simulink model "Enceinte_climatique_sans_correcteur"  (R2025b)
settings: Solver=VariableStepAuto  StartTime=0.0  StopTime=6  RelTol=1e-3
settings Model: Creator=boiteth  LastModifiedBy=rofte

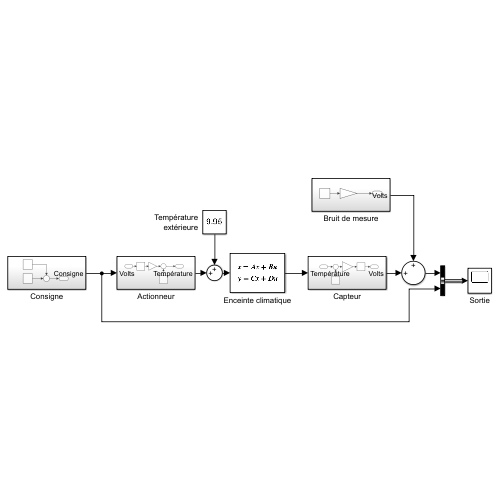
[thumbnail: Simulink's stored preview of the top-level diagram]
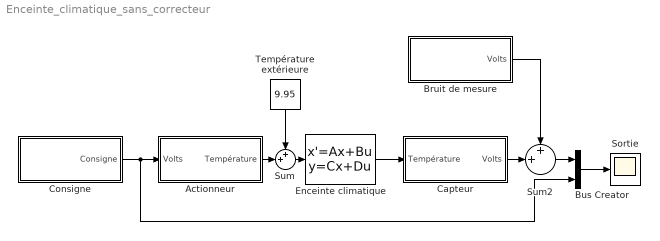
== system Enceinte_climatique_sans_correcteur ==
  Actionneur : Subsystem
  Bruit de mesure : Subsystem
  Bus Creator : BusCreator  Inputs=2
  Capteur : Subsystem
  Consigne : Subsystem
  Enceinte climatique : StateSpace  A=-2  B=2  D=0  InitialCondition=9.95
  Sortie : Scope
      settings: ActiveDisplayYMinimum=-1.1878376392458172  ActiveDisplayYMaximum=6.29146135794454
  Sum : Sum  Inputs=++|
  Sum2 : Sum  Inputs=++|
  Température extérieure : Constant  Value=9.95
  wires:
  Bus Creator/1 -> Sortie/1
  Consigne/1(Consigne) -> Actionneur/1(Volts), Bus Creator/2
  Enceinte climatique/1 -> Capteur/1(Température)
  Actionneur/1(Température) -> Sum/2
  Sum/1 -> Enceinte climatique/1
  Température extérieure/1 -> Sum/1
  Bruit de mesure/1(Volts) -> Sum2/1
  Capteur/1(Volts) -> Sum2/2
  Sum2/1 -> Bus Creator/1

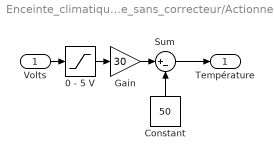
== system Enceinte_climatique_sans_correcteur/Actionneur ==
  Volts : Inport
  "0 - 5 V " : Saturate  UpperLimit=5  LowerLimit=0
  Constant : Constant  Value=50
  Gain : Gain  Gain=30
  Sum : Sum  Inputs=|+-
  Température : Outport
  wires:
  Volts/1 -> "0 - 5 V "/1
  "0 - 5 V "/1 -> Gain/1
  Gain/1 -> Sum/1
  Constant/1 -> Sum/2
  Sum/1 -> Température/1

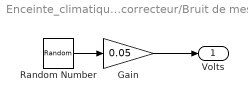
== system Enceinte_climatique_sans_correcteur/Bruit de mesure ==
  Gain : Gain  Gain=0.05
  Random Number : RandomNumber  Variance=0.5  SampleTime=0.01
  Volts : Outport
  wires:
  Random Number/1 -> Gain/1
  Gain/1 -> Volts/1

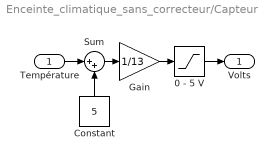
== system Enceinte_climatique_sans_correcteur/Capteur ==
  Température : Inport
  "0 - 5 V " : Saturate  UpperLimit=5  LowerLimit=0
  Constant : Constant  Value=5
  Gain : Gain  Gain=1/13
  Sum : Sum  Inputs=|++
  Volts : Outport
  wires:
  Constant/1 -> Sum/2
  Température/1 -> Sum/1
  Sum/1 -> Gain/1
  Gain/1 -> "0 - 5 V "/1
  "0 - 5 V "/1 -> Volts/1

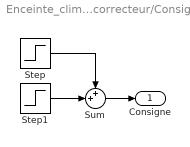
== system Enceinte_climatique_sans_correcteur/Consigne ==
  Step : Step  Time=4  After=-0.5  SampleTime=0
  Step1 : Step  Time=0.5  Before=1.66  After=2.33  SampleTime=0
  Sum : Sum  Inputs=++|
  Consigne : Outport
  wires:
  Step/1 -> Sum/1
  Step1/1 -> Sum/2
  Sum/1 -> Consigne/1
